simulink model "drone_2D_ode"  (R2020a)
settings: Solver=FixedStepAuto  StartTime=0.0  StopTime=10.0  RelTol=1e-3
values from neighbouring files (symbols this model uses):
  C_Dx = 0.2    [PID_design_setup.m]    (also in flight_controller_payload_setup.m)
  C_Dz = 0.2    [PID_design_setup.m]    (also in flight_controller_payload_setup.m)
  g = -9.81    [PID_design_setup.m]    (also in flight_controller_payload_setup.m)
  I_yy = 0.235    [PID_design_setup.m]    (also in flight_controller_payload_setup.m)
  M = 4.5    [PID_design_setup.m]    (also in flight_controller_payload_setup.m)
  r = 0.49*1/sqrt(2)    [PID_design_setup.m]    (also in flight_controller_payload_setup.m)
  rho = 1.225    [PID_design_setup.m]    (also in flight_controller_payload_setup.m)
  tau = 0.07    [PID_design_setup.m]    (also in flight_controller_payload_setup.m)
  u0 = -0.5*(M+m)*g*[1; 1]    [flight_controller_payload_setup.m]
  x0 = zeros(nx,1)    [flight_controller_payload_setup.m]    (also in flight_controller_setup.m = zeros(6,1))
settings Model: Creator=murray  LastModifiedBy=murray

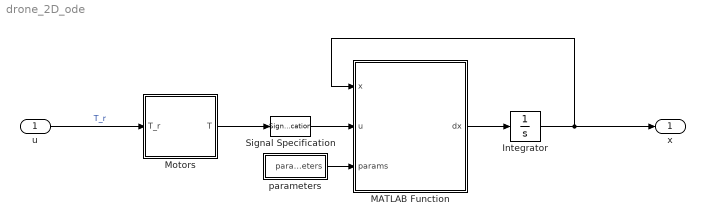
== system drone_2D_ode ==
  u : Inport  PortDimensions=[2, 1]
  Integrator : Integrator  InitialCondition=x0
  MATLAB Function : MATLAB Function  TreatAsAtomicUnit=on
  Motors : Subsystem
  Signal Specification : SignalSpecification  Dimensions=2
  parameters : Subsystem
  x : Outport
  wires:
  MATLAB Function/1(dx) -> Integrator/1
  Integrator/1 -> x/1, MATLAB Function/1(x)
  Signal Specification/1 -> MATLAB Function/2(u)
  parameters/1(parameters) -> MATLAB Function/3(params)
  u/1 -> Motors/1(T_r)  "T_r"
  Motors/1(T) -> Signal Specification/1

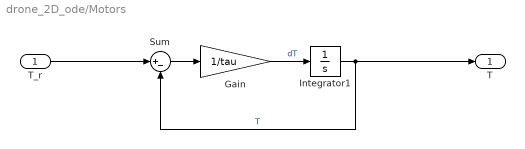
== system drone_2D_ode/Motors ==
  T_r : Inport
  Gain : Gain  Gain=1/tau
  Integrator1 : Integrator  InitialCondition=u0
  Sum : Sum  Inputs=|+-
  T : Outport
  wires:
  Sum/1 -> Gain/1
  Gain/1 -> Integrator1/1  "dT"
  Integrator1/1 -> T/1, Sum/2  "T"
  T_r/1 -> Sum/1

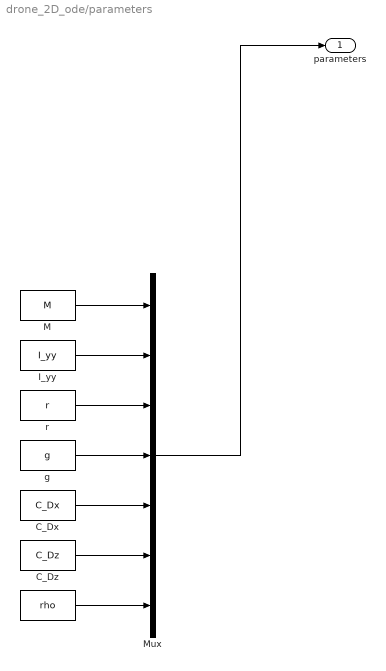
== system drone_2D_ode/parameters ==
  " " : Constant  Value=rho
  C_Dx : Constant  Value=C_Dx
  C_Dz : Constant  Value=C_Dz
  I_yy : Constant  Value=I_yy
  M : Constant  Value=M
  Mux : Mux  Inputs=7
  g : Constant  Value=g
  r : Constant  Value=r
  parameters : Outport
  wires:
  I_yy/1 -> Mux/2
  r/1 -> Mux/3
  Mux/1 -> parameters/1
  M/1 -> Mux/1
  C_Dx/1 -> Mux/5
  C_Dz/1 -> Mux/6
  g/1 -> Mux/4
  " "/1 -> Mux/7

== matlab function drone_2D_ode/MATLAB Function ==
  data: x input; u input; dx output; params input
function dx = drone_2D(x,u,params)
    %% Differential equations for drone in 2D without a payload
    % dx: x_dot, time derivative of state vector
    % x: state vector [x, z, theta]
    % u: input vector
    % params: parameters for drone model
    
    % Parameters:
    M = params(1); % Mass of drone body (at fulcrum)
    I_yy = params(2); % Moment of inertia of drone body
    r = params(3); % Distance from each rot`or force to COM of drone
    g = params(4); % Acceleration due to gravity (always negative)
    C_Dx = params(5); % Damping coef. of drone through air in x direction (f = cx*xdot)
    C_Dz = params(6); % Damping coef. of drone in z direction (f = cy*zdot)
    rho = params(7); % Air density
    
    % States (extract notation so we can copy over from symbolic toolbox equations)
    X1 = x(1);
    X2 = x(2);
    X3 = x(3);
    X4 = x(4);
    X5 = x(5);
    X6 = x(6);
    
    % Inputs
    T1 = u(1);
    T2 = u(2);
    
    % System equations
    dx = zeros(6,1);
    
    dx(1,1) = x(4);
    dx(2,1) = x(5);
    dx(3,1) = x(6);
    
    dx(4,1) = -(2*T1*sin(X3) + 2*T2*sin(X3) + C_Dx*X4*rho*abs(X4))/(2*M);
    dx(5,1) = -(2*M*g + 2*T1*cos(X3) + 2*T2*cos(X3) + C_Dz*X5*rho*abs(X5))/(2*M);
    dx(6,1) = -(T1*r - T2*r)/I_yy;

end
